simulink model "simulink_sin_PI"  (R2025b)
settings: Solver=VariableStepAuto  StartTime=0.0  StopTime=10.0  RelTol=1e-3
values from neighbouring files (symbols this model uses):
  CF = [0.05 0; 0 0]    [force_control.m]
  fd = [10; 0]    [force_control.m]    (also in force_control_params.m)
  K = [1000 0; 0 0]    [force_control.m]    (also in force_control_params.m)
  KD = [5000 0; 0 5000]    [force_control.m]    (also in force_control_params.m)
  KP = [5000 0; 0 5000]    [force_control.m]    (also in force_control_params.m)
  Md_inv = inv(Md)    [force_control.m]    (also in force_control_params.m)
  x_dot_initial = [0; 0]    [force_control.m]    (also in force_control_params.m)
  x_initial = [1.3; 0.7]    [force_control.m]    (also in force_control_params.m)
  xr = [1.2; 0.7]    [force_control.m]    (also in force_control_params.m)
settings Model: Creator=ruben  LastModifiedBy=ruben

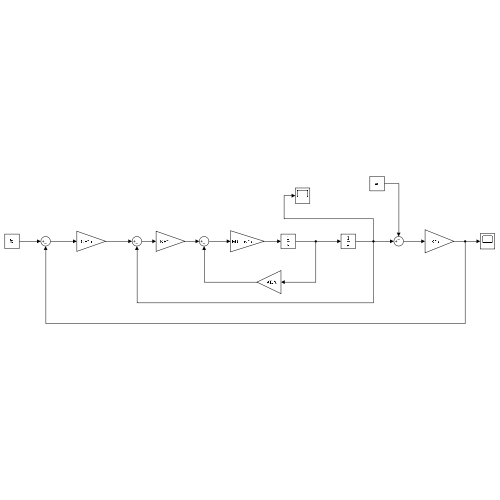
[thumbnail: Simulink's stored preview of the top-level diagram]
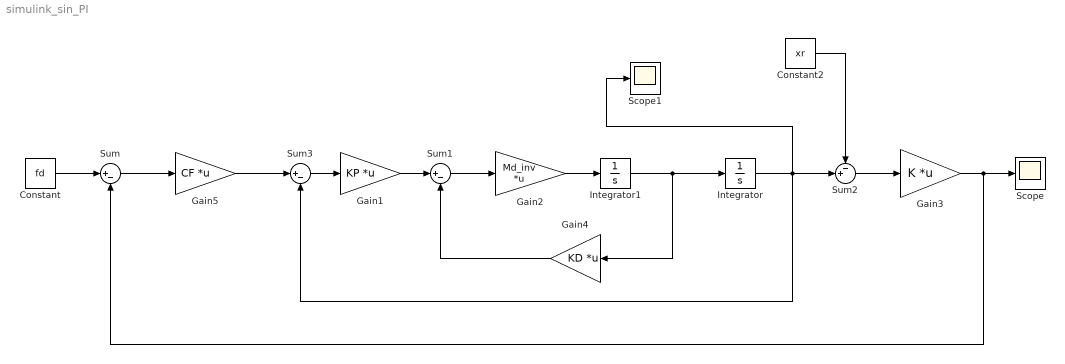
== system simulink_sin_PI ==
  Constant : Constant  Value=fd
  Constant2 : Constant  Value=xr
  Gain1 : Gain  Gain=KP  Multiplication=Matrix(K*u)
  Gain2 : Gain  Gain=Md_inv  Multiplication=Matrix(K*u)
  Gain3 : Gain  Gain=K  Multiplication=Matrix(K*u)
  Gain4 : Gain  Gain=KD  Multiplication=Matrix(K*u)
  Gain5 : Gain  Gain=CF  Multiplication=Matrix(K*u)
  Integrator : Integrator  InitialCondition=x_initial
  Integrator1 : Integrator  InitialCondition=x_dot_initial
  Scope : Scope
      settings: ActiveDisplayYMinimum=-127.22522986992354  ActiveDisplayYMaximum=125.24724776332494
  Scope1 : Scope
      settings: ActiveDisplayYMinimum=-0.16249873106547588  ActiveDisplayYMaximum=1.4624998590072753
  Sum : Sum  Inputs=|+-
  Sum1 : Sum  Inputs=|+-
  Sum2 : Sum  Inputs=-+|
  Sum3 : Sum  Inputs=|+-
  wires:
  Constant/1 -> Sum/1
  Sum3/1 -> Gain1/1
  Gain1/1 -> Sum1/1
  Sum1/1 -> Gain2/1
  Gain2/1 -> Integrator1/1
  Integrator1/1 -> Gain4/1, Integrator/1
  Sum2/1 -> Gain3/1
  Constant2/1 -> Sum2/1
  Gain3/1 -> Scope/1, Sum/2
  Gain4/1 -> Sum1/2
  Integrator/1 -> Scope1/1, Sum3/2, Sum2/2
  Sum/1 -> Gain5/1
  Gain5/1 -> Sum3/1
